simulink model "SEM_simulink"  (R2025b)
settings: Solver=VariableStepAuto  StartTime=0.0  StopTime=5  RelTol=1e-3
settings Model: Creator=leona  LastModifiedBy=leona

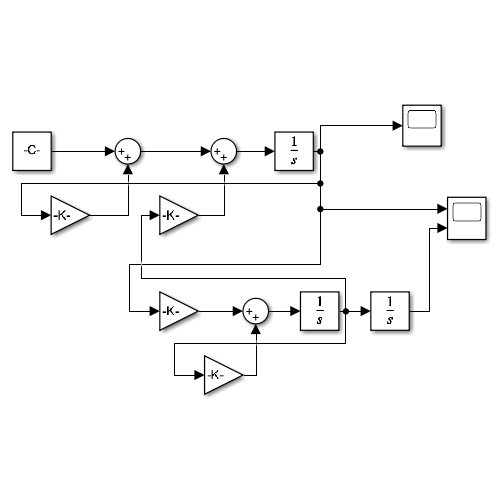
[thumbnail: Simulink's stored preview of the top-level diagram]
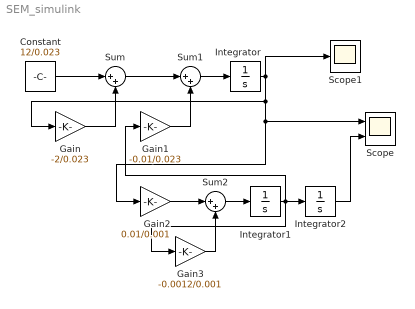
== system SEM_simulink ==
  Constant : Constant  Value=12/0.023
  Gain : Gain  Gain=-2/0.023
  Gain1 : Gain  Gain=-0.01/0.023
  Gain2 : Gain  Gain=0.01/0.001
  Gain3 : Gain  Gain=-0.0012/0.001
  Integrator : Integrator
  Integrator1 : Integrator
  Integrator2 : Integrator
  Scope : Scope  NumInputPorts=2
      settings: ActiveDisplayYMinimum=-25.143121448173787  ActiveDisplayYMaximum=226.28809303356414
  Scope1 : Scope
      settings: ActiveDisplayYMinimum=4.4417969455341053  ActiveDisplayYMaximum=6.56252486548639
  Sum : Sum  Inputs=|++
  Sum1 : Sum  Inputs=|++
  Sum2 : Sum  Inputs=|++
  wires:
  Constant/1 -> Sum/1
  Gain/1 -> Sum/2
  Sum/1 -> Sum1/1
  Gain1/1 -> Sum1/2
  Sum1/1 -> Integrator/1
  Integrator/1 -> Scope1/1, Gain2/1, Scope/1, Gain/1
  Gain2/1 -> Sum2/1
  Gain3/1 -> Sum2/2
  Sum2/1 -> Integrator1/1
  Integrator1/1 -> Gain3/1, Integrator2/1, Gain1/1
  Integrator2/1 -> Scope/2
